simulink model "Robot_Dog_with_equation"  (R2020a)
settings: Solver=VariableStepAuto  StartTime=0.0  StopTime=10.0  RelTol=1e-3
undefined symbols (not defined in the file): Levenberg, Marquardt, sigbuilder_block, X, Y, Z
libraries: sm_lib x93, nesl_utility x30, robotcorelib x2, robotmaniplib x2, sldrtlib x1
(part 3 of 3)

== system Robot_Dog_with_equation/Leg4/Base ==
  base : sm_lib/Body Elements/Cylindrical Solid  GraphicAmbientColor=[0.15 0.15 0.15 1.0]  BasedOnType=Density  CenterOfMass=[0 0 0]  CenterOfMassUnits=m  GraphicDiffuseColor=[0.5 0.5 0.5]  CylinderLength=0.1  CylinderLengthUnits=m  CylinderRadius=0.05  CylinderRadiusUnits=m  Density=1000  DensityUnits=kg/m^3  DoExposeReferenceFrame=on  GraphicEmissiveColor=[0.0 0.0 0.0 1.0]  ExportEntireGeometry=off  SerializedFrames=<Frames/>  MarkerShape=Sphere  MarkerSize=10  GraphicType=FromGeometry  InertiaType=CalculateFromGeometry  Mass=1  MassUnits=kg  MomentsOfInertia=[1 1 1]  MomentsOfInertiaUnits=kg*m^2  GraphicOpacity=1.0  ProductsOfInertia=[0 0 0]  ProductsOfInertiaUnits=kg*m^2  GraphicShininess=75  GraphicSpecularColor=[0.5 0.5 0.5 1.0]  GraphicVisPropType=SimpleVisualProperties
  base-to-J1 : sm_lib/Frames and Transforms/Rigid Transform  TranslationMethod=Cartesian  TranslationStandardOffset=0  TranslationLengthUnit=m  TranslationStandardAxis=+Z  TranslationCartesianOffset=[0 0 0]  TranslationROffset=0  TranslationROffsetUnits=m  TranslationZOffset=0  TranslationZOffsetUnits=m  TranslationThetaOffset=0  TranslationThetaOffsetUnits=deg  RotationMethod=StandardAxis  RotationAngleUnits=deg  RotationStandardAxis=+Z  RotationAngle=0  RotationArbitraryAxis=[0 0 1]  FollAlignAxisA=+X  BaseAlignAxisA=+Y  FollAlignAxisB=+Y  BaseAlignAxisB=+Z  RotationSequenceAxes=FollowerAxes  RotationSequence=XYX  RotationSequenceAngles=[0 0 0]  RotationSequenceAnglesUnits=deg  RotationMatrix=[1 0 0; 0 1 0; 0 0 1]
  world frame to base : sm_lib/Frames and Transforms/Rigid Transform  TranslationMethod=Cartesian  TranslationStandardOffset=0  TranslationLengthUnit=m  TranslationStandardAxis=+Z  TranslationCartesianOffset=[0 -.2 0]  TranslationROffset=0  TranslationROffsetUnits=m  TranslationZOffset=0  TranslationZOffsetUnits=m  TranslationThetaOffset=0  TranslationThetaOffsetUnits=deg  RotationMethod=StandardAxis  RotationAngleUnits=deg  RotationStandardAxis=+Y  RotationAngle=90  RotationArbitraryAxis=[0 0 1]  FollAlignAxisA=+X  BaseAlignAxisA=+Y  FollAlignAxisB=+Y  BaseAlignAxisB=+Z  RotationSequenceAxes=FollowerAxes  RotationSequence=XYX  RotationSequenceAngles=[0 0 0]  RotationSequenceAnglesUnits=deg  RotationMatrix=[1 0 0; 0 1 0; 0 0 1]
  J1 : PMIOPort  Side=Right
  "world frame " : PMIOPort  Port=2  Side=Left
  connections:
  world frame to base/LConn1 -- "world frame "/RConn1
  J1/RConn1 -- base-to-J1/RConn1
  base/RConn1 -- world frame to base/RConn1 -- base-to-J1/LConn1

== system Robot_Dog_with_equation/Leg4/EE ==
  Jee-to-ee : sm_lib/Frames and Transforms/Rigid Transform  TranslationMethod=Cartesian  TranslationStandardOffset=0  TranslationLengthUnit=m  TranslationStandardAxis=+Z  TranslationCartesianOffset=[0 0.01 0]  TranslationROffset=0  TranslationROffsetUnits=m  TranslationZOffset=0  TranslationZOffsetUnits=m  TranslationThetaOffset=0  TranslationThetaOffsetUnits=deg  RotationMethod=None  RotationAngleUnits=deg  RotationStandardAxis=+Z  RotationAngle=0.0  RotationArbitraryAxis=[0 0 1]  FollAlignAxisA=+X  BaseAlignAxisA=+Y  FollAlignAxisB=+Y  BaseAlignAxisB=+Z  RotationSequenceAxes=FollowerAxes  RotationSequence=XYX  RotationSequenceAngles=[0 0 0]  RotationSequenceAnglesUnits=deg  RotationMatrix=[1 0 0; 0 1 0; 0 0 1]
  ee : sm_lib/Body Elements/Brick Solid  GraphicAmbientColor=[0.15 0.15 0.15 1.0]  BasedOnType=Density  BrickDimensions=[0.02 0.02 0.02]  BrickDimensionUnits=m  CenterOfMass=[0 0 0]  CenterOfMassUnits=m  GraphicDiffuseColor=[0.2 1.0 0.0]  Density=1000  DensityUnits=kg/m^3  DoExposeReferenceFrame=on  GraphicEmissiveColor=[0.0 0.0 0.0 1.0]  ExportEntireGeometry=off  SerializedFrames=<Frames><Frame><Id>Frame1</Id><Value><Name>F1</Name><Origin><Source>ReferenceFrame</Source><FeatureName></FeatureName></Origin><PrimaryAxis><DefinedDirection>+Z</DefinedDirection><Source>ReferenceFrame</Source><SourceDirection>+Z</SourceDirection><FeatureName></FeatureName></PrimaryAxis><SecondaryAxis><DefinedDirection>+X</DefinedDirection><Source>ReferenceFrame</Source><SourceDirection>+X</SourceDirection><FeatureName></FeatureName></SecondaryAxis></Value></Frame><Frame><Id>Frame2</Id><Value><Name>F2</Name><Origin><Source>ReferenceFrame</Source><FeatureName></FeatureName></Origin><PrimaryAxis><DefinedDirection>+Z</DefinedDirection><Source>ReferenceFrame</Source><SourceDirection>+Z</SourceDirection><FeatureName></FeatureName></PrimaryAxis><SecondaryAxis><DefinedDirection>+X</DefinedDirection><Source>ReferenceFrame</Source><SourceDirection>+X</SourceDirection><FeatureName></FeatureName></SecondaryAxis></Value></Frame></Frames>  MarkerShape=Sphere  MarkerSize=10  GraphicType=FromGeometry  InertiaType=CalculateFromGeometry  Mass=1  MassUnits=kg  MomentsOfInertia=[1 1 1]  MomentsOfInertiaUnits=kg*m^2  GraphicOpacity=1.0  ProductsOfInertia=[0 0 0]  ProductsOfInertiaUnits=kg*m^2  GraphicShininess=75  GraphicSpecularColor=[0.5 0.5 0.5 1.0]  GraphicVisPropType=SimpleVisualProperties
  EE : PMIOPort  Side=Left
  connections:
  EE/RConn1 -- Jee-to-ee/LConn1
  Jee-to-ee/RConn1 -- ee/RConn1

== system Robot_Dog_with_equation/Leg4/Link1 ==
  base-to-J2 : sm_lib/Frames and Transforms/Rigid Transform  TranslationMethod=Cartesian  TranslationStandardOffset=0  TranslationLengthUnit=m  TranslationStandardAxis=+Z  TranslationCartesianOffset=[0 0 0.06]  TranslationROffset=0  TranslationROffsetUnits=m  TranslationZOffset=0  TranslationZOffsetUnits=m  TranslationThetaOffset=0  TranslationThetaOffsetUnits=deg  RotationMethod=StandardAxis  RotationAngleUnits=deg  RotationStandardAxis=-Z  RotationAngle=90  RotationArbitraryAxis=[0 0 1]  FollAlignAxisA=+X  BaseAlignAxisA=+Y  FollAlignAxisB=+Y  BaseAlignAxisB=+Z  RotationSequenceAxes=FollowerAxes  RotationSequence=XYX  RotationSequenceAngles=[0 0 0]  RotationSequenceAnglesUnits=deg  RotationMatrix=[1 0 0; 0 1 0; 0 0 1]
  base-to-J3 : sm_lib/Frames and Transforms/Rigid Transform  TranslationMethod=Cartesian  TranslationStandardOffset=0  TranslationLengthUnit=m  TranslationStandardAxis=+Z  TranslationCartesianOffset=[0 -0.05 0.05]  TranslationROffset=0  TranslationROffsetUnits=m  TranslationZOffset=0  TranslationZOffsetUnits=m  TranslationThetaOffset=0  TranslationThetaOffsetUnits=deg  RotationMethod=StandardAxis  RotationAngleUnits=deg  RotationStandardAxis=+X  RotationAngle=90  RotationArbitraryAxis=[0 0 1]  FollAlignAxisA=+X  BaseAlignAxisA=+Y  FollAlignAxisB=+Y  BaseAlignAxisB=+Z  RotationSequenceAxes=FollowerAxes  RotationSequence=XYX  RotationSequenceAngles=[0 0 0]  RotationSequenceAnglesUnits=deg  RotationMatrix=[1 0 0; 0 1 0; 0 0 1]
  base1 : sm_lib/Body Elements/Cylindrical Solid  GraphicAmbientColor=[0.15 0.15 0.15 1.0]  BasedOnType=Density  CenterOfMass=[0 0 0]  CenterOfMassUnits=m  GraphicDiffuseColor=[0.5 0.5 0.5]  CylinderLength=0.1  CylinderLengthUnits=m  CylinderRadius=0.05  CylinderRadiusUnits=m  Density=1000  DensityUnits=kg/m^3  DoExposeReferenceFrame=on  GraphicEmissiveColor=[0.0 0.0 0.0 1.0]  ExportEntireGeometry=off  SerializedFrames=<Frames/>  MarkerShape=Sphere  MarkerSize=10  GraphicType=FromGeometry  InertiaType=CalculateFromGeometry  Mass=1  MassUnits=kg  MomentsOfInertia=[1 1 1]  MomentsOfInertiaUnits=kg*m^2  GraphicOpacity=1.0  ProductsOfInertia=[0 0 0]  ProductsOfInertiaUnits=kg*m^2  GraphicShininess=75  GraphicSpecularColor=[0.5 0.5 0.5 1.0]  GraphicVisPropType=SimpleVisualProperties
  J2 : PMIOPort  Side=Right
  J1 : PMIOPort  Port=2  Side=Left
  connections:
  base1/RConn1 -- base-to-J2/LConn1 -- base-to-J3/RConn1
  base-to-J3/LConn1 -- J1/RConn1
  base-to-J2/RConn1 -- J2/RConn1

== system Robot_Dog_with_equation/Leg4/Link2 ==
  J1-to-Link1 : sm_lib/Frames and Transforms/Rigid Transform  TranslationMethod=Cartesian  TranslationStandardOffset=0  TranslationLengthUnit=m  TranslationStandardAxis=+Z  TranslationCartesianOffset=[0 0.15 0]  TranslationROffset=0  TranslationROffsetUnits=m  TranslationZOffset=0  TranslationZOffsetUnits=m  TranslationThetaOffset=0  TranslationThetaOffsetUnits=deg  RotationMethod=None  RotationAngleUnits=deg  RotationStandardAxis=+Z  RotationAngle=0.0  RotationArbitraryAxis=[0 0 1]  FollAlignAxisA=+X  BaseAlignAxisA=+Y  FollAlignAxisB=+Y  BaseAlignAxisB=+Z  RotationSequenceAxes=FollowerAxes  RotationSequence=XYX  RotationSequenceAngles=[0 0 0]  RotationSequenceAnglesUnits=deg  RotationMatrix=[1 0 0; 0 1 0; 0 0 1]
  Link1 : sm_lib/Body Elements/Brick Solid  GraphicAmbientColor=[0.15 0.15 0.15 1.0]  BasedOnType=Density  BrickDimensions=[0.02 0.3 0.02]  BrickDimensionUnits=m  CenterOfMass=[0 0 0]  CenterOfMassUnits=m  GraphicDiffuseColor=[0.5 0.5 0.5]  Density=1000  DensityUnits=kg/m^3  DoExposeReferenceFrame=on  GraphicEmissiveColor=[0.0 0.0 0.0 1.0]  ExportEntireGeometry=off  SerializedFrames=<Frames/>  MarkerShape=Sphere  MarkerSize=10  GraphicType=FromGeometry  InertiaType=CalculateFromGeometry  Mass=1  MassUnits=kg  MomentsOfInertia=[1 1 1]  MomentsOfInertiaUnits=kg*m^2  GraphicOpacity=1.0  ProductsOfInertia=[0 0 0]  ProductsOfInertiaUnits=kg*m^2  GraphicShininess=75  GraphicSpecularColor=[0.5 0.5 0.5 1.0]  GraphicVisPropType=SimpleVisualProperties
  Link1-to-J2 : sm_lib/Frames and Transforms/Rigid Transform  TranslationMethod=Cartesian  TranslationStandardOffset=0  TranslationLengthUnit=m  TranslationStandardAxis=+Z  TranslationCartesianOffset=[0 0.15 0]  TranslationROffset=0  TranslationROffsetUnits=m  TranslationZOffset=0  TranslationZOffsetUnits=m  TranslationThetaOffset=0  TranslationThetaOffsetUnits=deg  RotationMethod=None  RotationAngleUnits=deg  RotationStandardAxis=+Z  RotationAngle=0.0  RotationArbitraryAxis=[0 0 1]  FollAlignAxisA=+X  BaseAlignAxisA=+Y  FollAlignAxisB=+Y  BaseAlignAxisB=+Z  RotationSequenceAxes=FollowerAxes  RotationSequence=XYX  RotationSequenceAngles=[0 0 0]  RotationSequenceAnglesUnits=deg  RotationMatrix=[1 0 0; 0 1 0; 0 0 1]
  J3 : PMIOPort  Side=Right
  J2 : PMIOPort  Port=2  Side=Left
  connections:
  J1-to-Link1/RConn1 -- Link1-to-J2/LConn1 -- Link1/RConn1
  J1-to-Link1/LConn1 -- J2/RConn1
  J3/RConn1 -- Link1-to-J2/RConn1

== system Robot_Dog_with_equation/Leg4/Link3 ==
  J3-to-Link3 : sm_lib/Frames and Transforms/Rigid Transform  TranslationMethod=Cartesian  TranslationStandardOffset=0  TranslationLengthUnit=m  TranslationStandardAxis=+Z  TranslationCartesianOffset=[0 0.15 0]  TranslationROffset=0  TranslationROffsetUnits=m  TranslationZOffset=0  TranslationZOffsetUnits=m  TranslationThetaOffset=0  TranslationThetaOffsetUnits=deg  RotationMethod=None  RotationAngleUnits=deg  RotationStandardAxis=+Z  RotationAngle=0.0  RotationArbitraryAxis=[0 0 1]  FollAlignAxisA=+X  BaseAlignAxisA=+Y  FollAlignAxisB=+Y  BaseAlignAxisB=+Z  RotationSequenceAxes=FollowerAxes  RotationSequence=XYX  RotationSequenceAngles=[0 0 0]  RotationSequenceAnglesUnits=deg  RotationMatrix=[1 0 0; 0 1 0; 0 0 1]
  Link3 : sm_lib/Body Elements/Brick Solid  GraphicAmbientColor=[0.15 0.15 0.15 1.0]  BasedOnType=Density  BrickDimensions=[0.02 0.3 0.02]  BrickDimensionUnits=m  CenterOfMass=[0 0 0]  CenterOfMassUnits=m  GraphicDiffuseColor=[0.2 0.2 1.0]  Density=1000  DensityUnits=kg/m^3  DoExposeReferenceFrame=on  GraphicEmissiveColor=[0.0 0.0 0.0 1.0]  ExportEntireGeometry=off  SerializedFrames=<Frames/>  MarkerShape=Sphere  MarkerSize=10  GraphicType=FromGeometry  InertiaType=CalculateFromGeometry  Mass=1  MassUnits=kg  MomentsOfInertia=[1 1 1]  MomentsOfInertiaUnits=kg*m^2  GraphicOpacity=1.0  ProductsOfInertia=[0 0 0]  ProductsOfInertiaUnits=kg*m^2  GraphicShininess=75  GraphicSpecularColor=[0.5 0.5 0.5 1.0]  GraphicVisPropType=SimpleVisualProperties
  Link3-to-Jee : sm_lib/Frames and Transforms/Rigid Transform  TranslationMethod=Cartesian  TranslationStandardOffset=0  TranslationLengthUnit=m  TranslationStandardAxis=+Z  TranslationCartesianOffset=[0 0.15 0]  TranslationROffset=0  TranslationROffsetUnits=m  TranslationZOffset=0  TranslationZOffsetUnits=m  TranslationThetaOffset=0  TranslationThetaOffsetUnits=deg  RotationMethod=None  RotationAngleUnits=deg  RotationStandardAxis=+Z  RotationAngle=0.0  RotationArbitraryAxis=[0 0 1]  FollAlignAxisA=+X  BaseAlignAxisA=+Y  FollAlignAxisB=+Y  BaseAlignAxisB=+Z  RotationSequenceAxes=FollowerAxes  RotationSequence=XYX  RotationSequenceAngles=[0 0 0]  RotationSequenceAnglesUnits=deg  RotationMatrix=[1 0 0; 0 1 0; 0 0 1]
  Jee : PMIOPort  Side=Right
  J3 : PMIOPort  Port=2  Side=Left
  connections:
  Link3/RConn1 -- Link3-to-Jee/LConn1 -- J3-to-Link3/RConn1
  Link3-to-Jee/RConn1 -- Jee/RConn1
  J3-to-Link3/LConn1 -- J3/RConn1

== matlab function Robot_Dog_with_equation/Eq Leg1 ==
  data: x output; y output; z output; t input
function [x,y,z] = fcn(t)

T_track = 100;
f = 1/T_track;
w = 100 * pi * f;
%x = input('x = ');
y = -.1;%input('y = ');
%z = input('z = ');

    x = .1*cos(w*t)+.4;
    if x>.4
        x=.4;
    end
    z = .1*sin(w*t);

== matlab function Robot_Dog_with_equation/Inverse kinematic ==
  data: x input; y input; z input; q1 output; q2 output; q3 output
function [q1,q2,q3] = fcn(x,y,z)
%%
a2 = 0.3;
a3 = 0.32;
d2=0.1;

%%
s = x^2+y^2-d2^2;
if s<0 
   s=0;
end
q1 = atan2(y,x)+atan2(d2, sqrt(s));
%update xc and yc
D = (x^2+y^2-d2^2+z^2-a2^2-a3^2)/(2*a2*a3);
D1 = 1-D^2;
if D1<0
   D1=0;
end
q3 = atan2(-sqrt(D1),D);
h1 =atan2(a3*sin(q3),a2+(a3*cos(q3)));
h2 = atan2(z,sqrt(abs(x^2+y^2-d2^2)));
q2 = h2-h1;

== matlab function Robot_Dog_with_equation/Inverse kinematic3 ==
  data: x input; y input; z input; q1 output; q2 output; q3 output
function [q1,q2,q3] = fcn(x,y,z)
%%
a2 = 0.3;
a3 = 0.32;
d2=0.1;

%%
s = x^2+y^2-d2^2;
if s<0 
   s=0;
end
q1 = atan2(y,x)+atan2(d2, sqrt(s));
%update xc and yc
D = (x^2+y^2-d2^2+z^2-a2^2-a3^2)/(2*a2*a3);
D1 = 1-D^2;
if D1<0
   D1=0;
end
q3 = atan2(sqrt(D1),D);
h1 =atan2(a3*sin(q3),a2+(a3*cos(q3)));
h2 = atan2(z,sqrt(abs(x^2+y^2-d2^2)));
q2 = h2-h1;

== matlab function Robot_Dog_with_equation/ Eq Leg3 ==
  data: x output; y output; z output; t input
function [x,y,z] = fcn(t)

T_track = 100;
f = 1/T_track;
w = -100 * pi * f;
%x = input('x = ');
y = -.1;%input('y = ');
%z = input('z = ');

    x = .1*cos(w*t)+.4;
    if x>.4
        x=.4;
    end
    z = .1*sin(w*t);

== matlab function Robot_Dog_with_equation/Inverse kinematic2 ==
  data: x input; y input; z input; q1 output; q2 output; q3 output
function [q1,q2,q3] = fcn(x,y,z)
%%
a2 = 0.3;
a3 = 0.32;
d2=0.1;

%%
s = x^2+y^2-d2^2;
if s<0 
   s=0;
end
q1 = atan2(y,x)+atan2(d2, sqrt(s));
%update xc and yc
D = (x^2+y^2-d2^2+z^2-a2^2-a3^2)/(2*a2*a3);
D1 = 1-D^2;
if D1<0
   D1=0;
end
q3 = atan2(-sqrt(D1),D);
h1 =atan2(a3*sin(q3),a2+(a3*cos(q3)));
h2 = atan2(z,sqrt(abs(x^2+y^2-d2^2)));
q2 = h2-h1;

== matlab function Robot_Dog_with_equation/Eq Leg2 ==
  data: x output; y output; z output; t input
function [x,y,z] = fcn(t)

T_track = 100;
f = 1/T_track;
w = 100 * pi * f;
%x = input('x = ');
y = -.1;%input('y = ');
%z = input('z = ');

    x = .1*cos(w*t-pi)+.4;
    if x>.4
        x=.4;
    end
    z = .1*sin(w*t-pi);

== matlab function Robot_Dog_with_equation/Inverse kinematic 4 ==
  data: x input; y input; z input; q1 output; q2 output; q3 output
function [q1,q2,q3] = fcn(x,y,z)
%%
a2 = 0.3;
a3 = 0.32;
d2=0.1;

%%
s = x^2+y^2-d2^2;
if s<0 
   s=0;
end
q1 = atan2(y,x)+atan2(d2, sqrt(s));
%update xc and yc
D = (x^2+y^2-d2^2+z^2-a2^2-a3^2)/(2*a2*a3);
D1 = 1-D^2;
if D1<0
   D1=0;
end
q3 = atan2(sqrt(D1),D);
h1 =atan2(a3*sin(q3),a2+(a3*cos(q3)));
h2 = atan2(z,sqrt(abs(x^2+y^2-d2^2)));
q2 = h2-h1;

== matlab function Robot_Dog_with_equation/Eq Leg 4 ==
  data: x output; y output; z output; t input
function [x,y,z] = fcn(t)

T_track = 100;
f = 1/T_track;
w = -100 * pi * f;
%x = input('x = ');
y = -.1;%input('y = ');
%z = input('z = ');

    x = .1*cos(w*t-pi)+.4;
    if x>.4
        x=.4;
    end
    z = .1*sin(w*t-pi);
